simulink model "lab3_p6"  (R2020a)
settings: Solver=VariableStepAuto  StartTime=0.0  StopTime=stop_time  RelTol=1e-3
InitFcn:
  | % Read in the audio file
  | [input_wav_signal, Fs_in] = audioread('acoustic.wav');
  | % Fs_in = 11025, we need to convert this to Fs = 48k
  | 
  | % Convert the Sampling rate to 48 kHz
  | signal = resample(input_wav_signal, 48000, 11025);
  | Fs = 48000; % This is our desired sample rate that we converted to
  | Ts = 1/Fs; % The associated sample period
  | 
  | % Put signal inot a timeseries format
  | timevals = [0:length(signal)-1]*Ts;
  | input_signal = timeseries(signal,timevals);
  | 
  | % Set the simulation stop time
  | stop_time = length(signal)*Ts;
  | 
  | % Fixed-point precision we want the signal to be converted to
  | W_bits = 32;
  | F_bits = 28;
  | 
  | % Counter
  | max_counter_time = 5; % yime in seconds
  | max_reset_Nbits = ceil(log2(max_counter_time*Fs)); % size of counter
  | 
  | max_reset_time = 300; % time in milliseconds
  | max_reset_threshold = ceil(max_reset_time/1000 * Fs); % reset time in samples
  | 
  | % LED Persistence
  | LED_persistence_Nbits = 15;
  | LED_persistence_time = 100; %msec
  | LED_persistence = ceil(LED_persistence_time/1000 * Fs);
StopFcn:
  | y_out = output_signal.Data(:);
  | plot(y_out)
  | soundsc(y_out,Fs)
undefined symbols (not defined in the file): magnitude
libraries: hdlsllib x10, dspsrcs4 x2, simulink x1
settings Model: Creator=Owner  LastModifiedBy=Owner
settings DataIOCC: ReturnWorkspaceOutputs=off

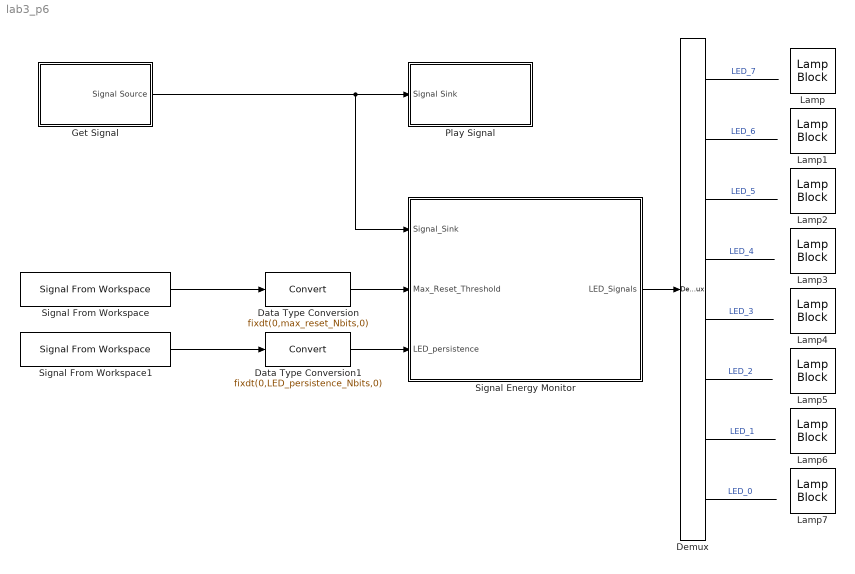
== system lab3_p6 ==
  Data Type Conversion : DataTypeConversion  OutDataTypeStr=fixdt(0,max_reset_Nbits,0)
  Data Type Conversion1 : DataTypeConversion  OutDataTypeStr=fixdt(0,LED_persistence_Nbits,0)
  Demux : Demux  Outputs=8
  Get Signal : Subsystem
  Lamp{,1..7} (8 alike) : LampBlock
  Play Signal : Subsystem
  Signal Energy Monitor : Subsystem
  Signal From Workspace : dspsrcs4/Signal From Workspace  X=max_reset_threshold  Ts=Ts  nsamps=1  OutputAfterFinalValue=Holding final value  ignoreOrWarnInputAndFrameLengths=off  OutputFrames=off
  Signal From Workspace1 : dspsrcs4/Signal From Workspace  X=LED_persistence  Ts=Ts  nsamps=1  OutputAfterFinalValue=Holding final value  ignoreOrWarnInputAndFrameLengths=off  OutputFrames=off
  wires:
  Get Signal/1(Signal Source) -> Signal Energy Monitor/1(Signal_Sink), Play Signal/1(Signal Sink)
  Signal Energy Monitor/1(LED_Signals) -> Demux/1
  Data Type Conversion/1 -> Signal Energy Monitor/2(Max_Reset_Threshold)
  Signal From Workspace/1 -> Data Type Conversion/1
  Demux/1 -> ?  "LED_7"
  Demux/2 -> ?  "LED_6"
  Demux/3 -> ?  "LED_5"
  Demux/4 -> ?  "LED_4"
  Demux/5 -> ?  "LED_3"
  Demux/6 -> ?  "LED_2"
  Demux/7 -> ?  "LED_1"
  Demux/8 -> ?  "LED_0"
  Signal From Workspace1/1 -> Data Type Conversion1/1
  Data Type Conversion1/1 -> Signal Energy Monitor/3(LED_persistence)

== system lab3_p6/Get Signal ==
  Data Type Conversion : DataTypeConversion  OutDataTypeStr=fixdt(1,W_bits,F_bits)
  From Workspace : FromWorkspace  VariableName=input_signal  SampleTime=Ts
  Signal Source : Outport
  wires:
  From Workspace/1 -> Data Type Conversion/1
  Data Type Conversion/1 -> Signal Source/1

== system lab3_p6/Play Signal ==
  Signal Sink : Inport
  Data Type Conversion1 : DataTypeConversion  OutDataTypeStr=double
  To Workspace : ToWorkspace  VariableName=output_signal  SaveFormat=Timeseries  SampleTime=-1
  wires:
  Data Type Conversion1/1 -> To Workspace/1
  Signal Sink/1 -> Data Type Conversion1/1

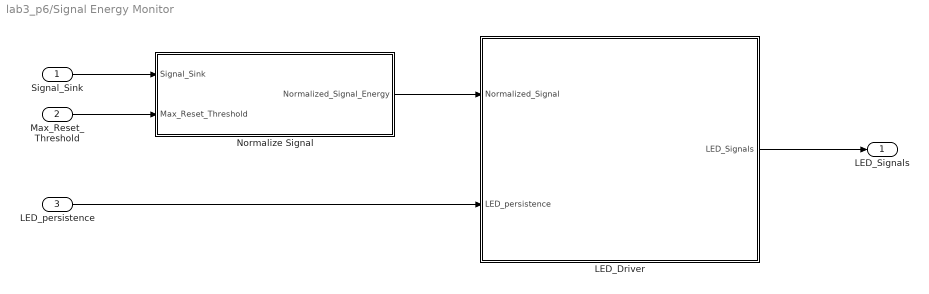
== system lab3_p6/Signal Energy Monitor ==
  Signal_Sink : Inport
  Max_Reset_Threshold : Inport  Port=2
  LED_persistence : Inport  Port=3
  LED_Driver : Subsystem
  Normalize Signal : Subsystem
  LED_Signals : Outport  VectorParamsAs1DForOutWhenUnconnected=off
  wires:
  Signal_Sink/1 -> Normalize Signal/1(Signal_Sink)
  Max_Reset_Threshold/1 -> Normalize Signal/2(Max_Reset_Threshold)
  Normalize Signal/1(Normalized_Signal_Energy) -> LED_Driver/1(Normalized_Signal)
  LED_Driver/1(LED_Signals) -> LED_Signals/1
  LED_persistence/1 -> LED_Driver/2(LED_persistence)

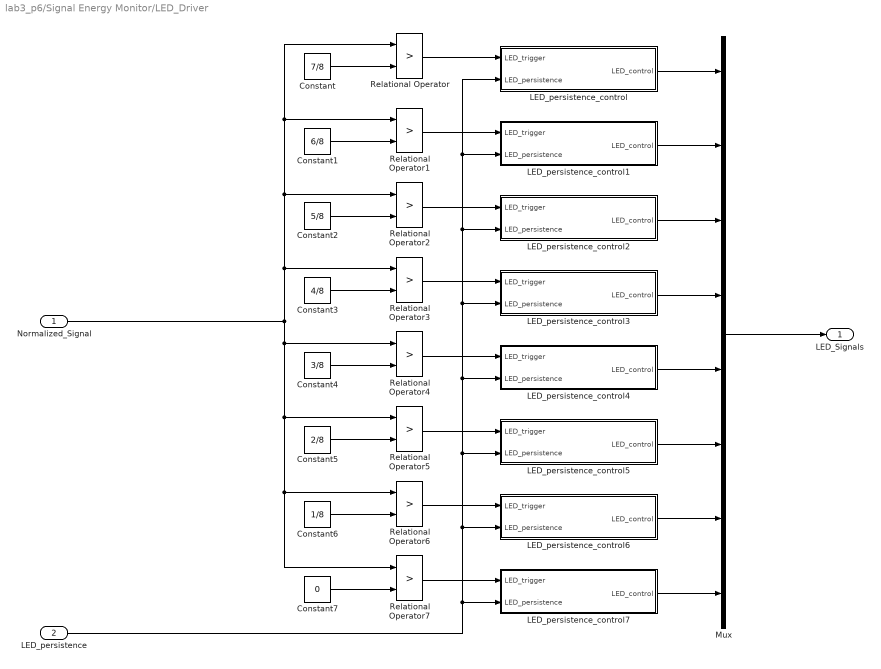
== system lab3_p6/Signal Energy Monitor/LED_Driver ==
  Normalized_Signal : Inport
  LED_persistence : Inport  Port=2
  Constant : Constant  Value=7/8  OutDataTypeStr=fixdt(1,W_bits,F_bits)  SampleTime=Ts
  Constant1 : Constant  Value=6/8  OutDataTypeStr=fixdt(1,W_bits,F_bits)  SampleTime=Ts
  Constant2 : Constant  Value=5/8  OutDataTypeStr=fixdt(1,W_bits,F_bits)  SampleTime=Ts
  Constant3 : Constant  Value=4/8  OutDataTypeStr=fixdt(1,W_bits,F_bits)  SampleTime=Ts
  Constant4 : Constant  Value=3/8  OutDataTypeStr=fixdt(1,W_bits,F_bits)  SampleTime=Ts
  Constant5 : Constant  Value=2/8  OutDataTypeStr=fixdt(1,W_bits,F_bits)  SampleTime=Ts
  Constant6 : Constant  Value=1/8  OutDataTypeStr=fixdt(1,W_bits,F_bits)  SampleTime=Ts
  Constant7 : Constant  Value=0  OutDataTypeStr=fixdt(1,W_bits,F_bits)  SampleTime=Ts
  LED_persistence_control : Subsystem
  LED_persistence_control1 : Subsystem
  LED_persistence_control2 : Subsystem
  LED_persistence_control3 : Subsystem
  LED_persistence_control4 : Subsystem
  LED_persistence_control5 : Subsystem
  LED_persistence_control6 : Subsystem
  LED_persistence_control7 : Subsystem
  Mux : Mux  Inputs=8
  Relational Operator{,1..7} (8 alike) : RelationalOperator  Operator=>  OutDataTypeStr=boolean  RndMeth=Nearest
  LED_Signals : Outport
  wires:
  Constant/1 -> Relational Operator/2
  Normalized_Signal/1 -> Relational Operator4/1, Relational Operator5/1, Relational Operator7/1, Relational Operator6/1, Relational Operator/1, Relational Operator1/1, Relational Operator2/1, Relational Operator3/1
  Constant1/1 -> Relational Operator1/2
  Constant2/1 -> Relational Operator2/2
  Constant3/1 -> Relational Operator3/2
  Constant4/1 -> Relational Operator4/2
  Constant5/1 -> Relational Operator5/2
  Constant6/1 -> Relational Operator6/2
  Constant7/1 -> Relational Operator7/2
  Mux/1 -> LED_Signals/1
  Relational Operator/1 -> LED_persistence_control/1(LED_trigger)
  LED_persistence_control/1(LED_control) -> Mux/1
  Relational Operator1/1 -> LED_persistence_control1/1(LED_trigger)
  Relational Operator2/1 -> LED_persistence_control2/1(LED_trigger)
  Relational Operator3/1 -> LED_persistence_control3/1(LED_trigger)
  Relational Operator4/1 -> LED_persistence_control4/1(LED_trigger)
  Relational Operator5/1 -> LED_persistence_control5/1(LED_trigger)
  LED_persistence/1 -> LED_persistence_control7/2(LED_persistence), LED_persistence_control6/2(LED_persistence), LED_persistence_control5/2(LED_persistence), LED_persistence_control4/2(LED_persistence), LED_persistence_control3/2(LED_persistence), LED_persistence_control2/2(LED_persistence), LED_persistence_control1/2(LED_persistence), LED_persistence_control/2(LED_persistence)
  Relational Operator6/1 -> LED_persistence_control6/1(LED_trigger)
  Relational Operator7/1 -> LED_persistence_control7/1(LED_trigger)
  LED_persistence_control7/1(LED_control) -> Mux/8
  LED_persistence_control6/1(LED_control) -> Mux/7
  LED_persistence_control5/1(LED_control) -> Mux/6
  LED_persistence_control4/1(LED_control) -> Mux/5
  LED_persistence_control3/1(LED_control) -> Mux/4
  LED_persistence_control2/1(LED_control) -> Mux/3
  LED_persistence_control1/1(LED_control) -> Mux/2

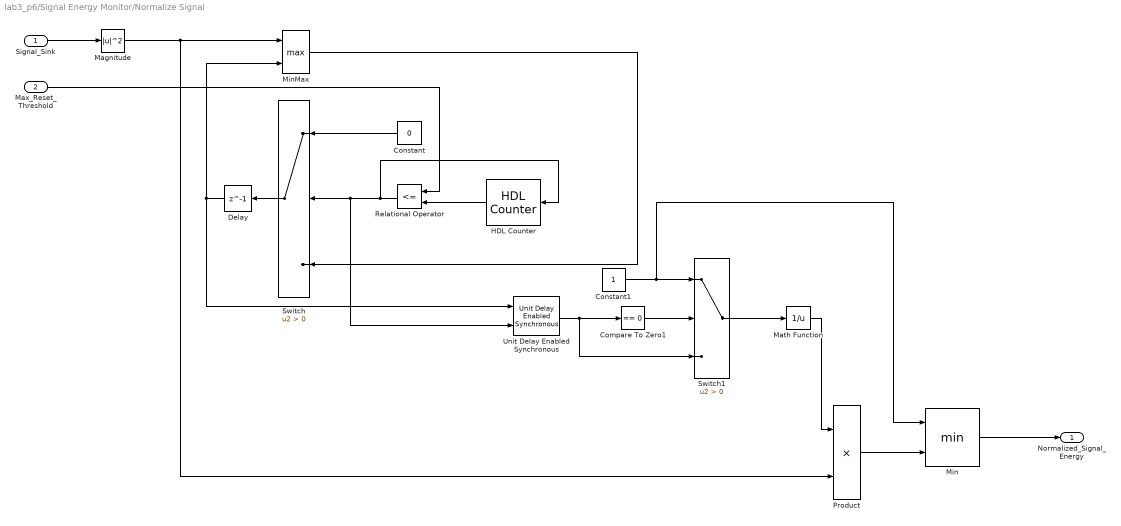
== system lab3_p6/Signal Energy Monitor/Normalize Signal ==
  Signal_Sink : Inport
  Max_Reset_Threshold : Inport  Port=2
  Compare To Zero1 : simulink/Logic and Bit Operations/Compare To Zero  relop===  OutDataTypeStr=boolean
  Constant : Constant  Value=0  OutDataTypeStr=fixdt(1,W_bits,F_bits)  SampleTime=Ts
  Constant1 : Constant  OutDataTypeStr=fixdt(1,W_bits,F_bits)  SampleTime=Ts
  Delay : Delay  DelayLength=1
  HDL Counter : hdlsllib/Sources/HDL Counter  CountType=Free running  CountInit=0  CountStep=1  CountMax=25  CountFromType=Initial value  CountFrom=0  CountResetPort=on  CountLoadPort=off  CountEnbPort=off  CountDirPort=off  CountDataType=Unsigned  CountWordLen=max_reset_Nbits  CountFracLen=0  CountSampTime=1
  Magnitude : Math  Operator=magnitude^2  SignedPower=on  RndMeth=Zero  SaturateOnIntegerOverflow=on
  Math Function : Math  Operator=reciprocal  OutDataTypeStr=fixdt(1,32,24)  SaturateOnIntegerOverflow=on
  Min : MinMax  Inputs=2  OutDataTypeStr=fixdt(1,W_bits,F_bits)
  MinMax : MinMax  Function=max  Inputs=2
  Product : Product  OutDataTypeStr=fixdt(1,W_bits,F_bits)
  Relational Operator : RelationalOperator  Operator=<=  OutDataTypeStr=boolean  RndMeth=Nearest
  Switch : Switch  Criteria=u2 > Threshold
  Switch1 : Switch  Criteria=u2 > Threshold
  Unit Delay Enabled Synchronous : hdlsllib/Discrete/Unit Delay Enabled Synchronous  InitialCondition=0.0  SampleTime=-1
      settings: SourceProductBaseCode=SL
  Normalized_Signal_Energy : Outport
  wires:
  Delay/1 -> MinMax/2, Unit Delay Enabled Synchronous/1
  Unit Delay Enabled Synchronous/1 -> Switch1/3, Compare To Zero1/1
  Min/1 -> Normalized_Signal_Energy/1
  Math Function/1 -> Product/1
  Relational Operator/1 -> HDL Counter/1, Unit Delay Enabled Synchronous/2, Switch/2
  Constant/1 -> Switch/1
  MinMax/1 -> Switch/3
  Constant1/1 -> Min/1, Switch1/1
  Compare To Zero1/1 -> Switch1/2
  Magnitude/1 -> Product/2, MinMax/1
  Switch/1 -> Delay/1
  Signal_Sink/1 -> Magnitude/1
  Switch1/1 -> Math Function/1
  Product/1 -> Min/2
  HDL Counter/1 -> Relational Operator/2
  Max_Reset_Threshold/1 -> Relational Operator/1

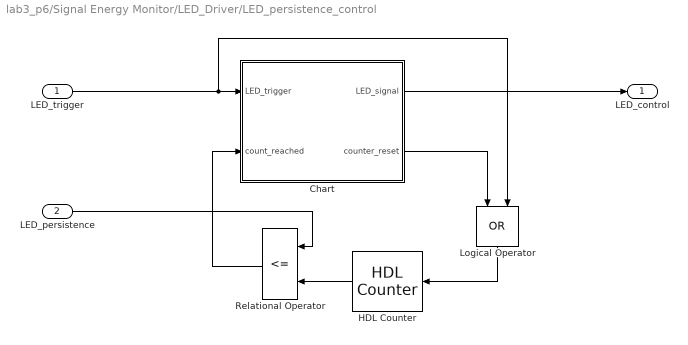
== system lab3_p6/Signal Energy Monitor/LED_Driver/LED_persistence_control ==
  LED_trigger : Inport
  LED_persistence : Inport  Port=2
  Chart : Stateflow chart  TreatAsAtomicUnit=on
  HDL Counter : hdlsllib/Sources/HDL Counter  CountType=Free running  CountInit=0  CountStep=1  CountMax=25  CountFromType=Initial value  CountFrom=0  CountResetPort=on  CountLoadPort=off  CountEnbPort=off  CountDirPort=off  CountDataType=Unsigned  CountWordLen=LED_persistence_Nbits  CountFracLen=0  CountSampTime=1
  Logical Operator : Logic  Operator=OR  AllPortsSameDT=off  OutDataTypeStr=boolean
  Relational Operator : RelationalOperator  Operator=<=  OutDataTypeStr=boolean  RndMeth=Nearest
  LED_control : Outport
  wires:
  LED_trigger/1 -> Logical Operator/2, Chart/1(LED_trigger)
  Logical Operator/1 -> HDL Counter/1
  Chart/2(counter_reset) -> Logical Operator/1
  LED_persistence/1 -> Relational Operator/1
  HDL Counter/1 -> Relational Operator/2
  Relational Operator/1 -> Chart/2(count_reached)
  Chart/1(LED_signal) -> LED_control/1

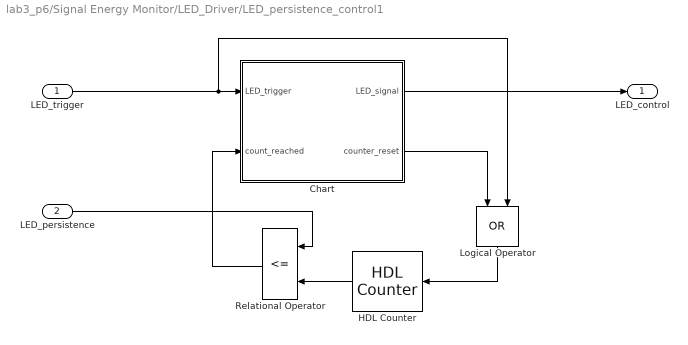
== system lab3_p6/Signal Energy Monitor/LED_Driver/LED_persistence_control1 ==
  LED_trigger : Inport
  LED_persistence : Inport  Port=2
  Chart : Stateflow chart  TreatAsAtomicUnit=on
  HDL Counter : hdlsllib/Sources/HDL Counter  CountType=Free running  CountInit=0  CountStep=1  CountMax=25  CountFromType=Initial value  CountFrom=0  CountResetPort=on  CountLoadPort=off  CountEnbPort=off  CountDirPort=off  CountDataType=Unsigned  CountWordLen=LED_persistence_Nbits  CountFracLen=0  CountSampTime=1
  Logical Operator : Logic  Operator=OR  AllPortsSameDT=off  OutDataTypeStr=boolean
  Relational Operator : RelationalOperator  Operator=<=  OutDataTypeStr=boolean  RndMeth=Nearest
  LED_control : Outport
  wires:
  LED_trigger/1 -> Logical Operator/2, Chart/1(LED_trigger)
  Logical Operator/1 -> HDL Counter/1
  Chart/2(counter_reset) -> Logical Operator/1
  LED_persistence/1 -> Relational Operator/1
  HDL Counter/1 -> Relational Operator/2
  Relational Operator/1 -> Chart/2(count_reached)
  Chart/1(LED_signal) -> LED_control/1

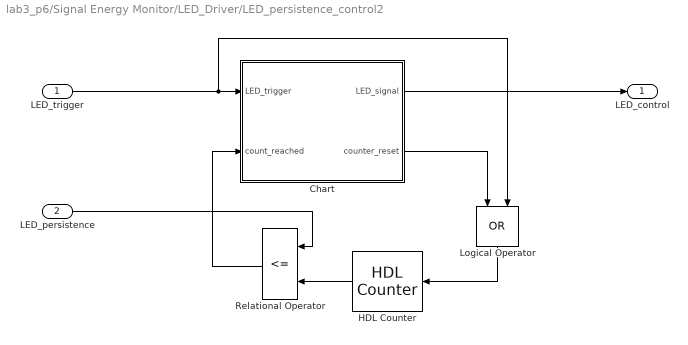
== system lab3_p6/Signal Energy Monitor/LED_Driver/LED_persistence_control2 ==
  LED_trigger : Inport
  LED_persistence : Inport  Port=2
  Chart : Stateflow chart  TreatAsAtomicUnit=on
  HDL Counter : hdlsllib/Sources/HDL Counter  CountType=Free running  CountInit=0  CountStep=1  CountMax=25  CountFromType=Initial value  CountFrom=0  CountResetPort=on  CountLoadPort=off  CountEnbPort=off  CountDirPort=off  CountDataType=Unsigned  CountWordLen=LED_persistence_Nbits  CountFracLen=0  CountSampTime=1
  Logical Operator : Logic  Operator=OR  AllPortsSameDT=off  OutDataTypeStr=boolean
  Relational Operator : RelationalOperator  Operator=<=  OutDataTypeStr=boolean  RndMeth=Nearest
  LED_control : Outport
  wires:
  LED_trigger/1 -> Logical Operator/2, Chart/1(LED_trigger)
  Logical Operator/1 -> HDL Counter/1
  Chart/2(counter_reset) -> Logical Operator/1
  LED_persistence/1 -> Relational Operator/1
  HDL Counter/1 -> Relational Operator/2
  Relational Operator/1 -> Chart/2(count_reached)
  Chart/1(LED_signal) -> LED_control/1

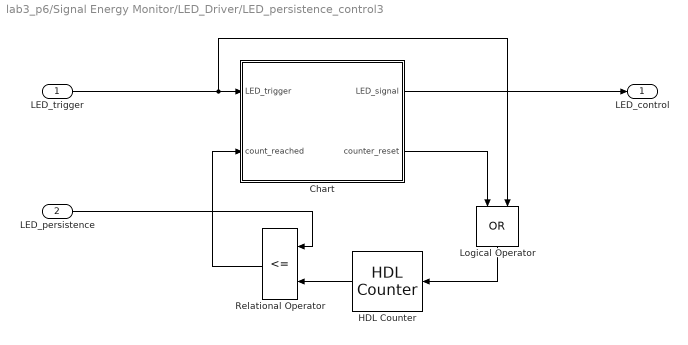
== system lab3_p6/Signal Energy Monitor/LED_Driver/LED_persistence_control3 ==
  LED_trigger : Inport
  LED_persistence : Inport  Port=2
  Chart : Stateflow chart  TreatAsAtomicUnit=on
  HDL Counter : hdlsllib/Sources/HDL Counter  CountType=Free running  CountInit=0  CountStep=1  CountMax=25  CountFromType=Initial value  CountFrom=0  CountResetPort=on  CountLoadPort=off  CountEnbPort=off  CountDirPort=off  CountDataType=Unsigned  CountWordLen=LED_persistence_Nbits  CountFracLen=0  CountSampTime=1
  Logical Operator : Logic  Operator=OR  AllPortsSameDT=off  OutDataTypeStr=boolean
  Relational Operator : RelationalOperator  Operator=<=  OutDataTypeStr=boolean  RndMeth=Nearest
  LED_control : Outport
  wires:
  LED_trigger/1 -> Logical Operator/2, Chart/1(LED_trigger)
  Logical Operator/1 -> HDL Counter/1
  Chart/2(counter_reset) -> Logical Operator/1
  LED_persistence/1 -> Relational Operator/1
  HDL Counter/1 -> Relational Operator/2
  Relational Operator/1 -> Chart/2(count_reached)
  Chart/1(LED_signal) -> LED_control/1

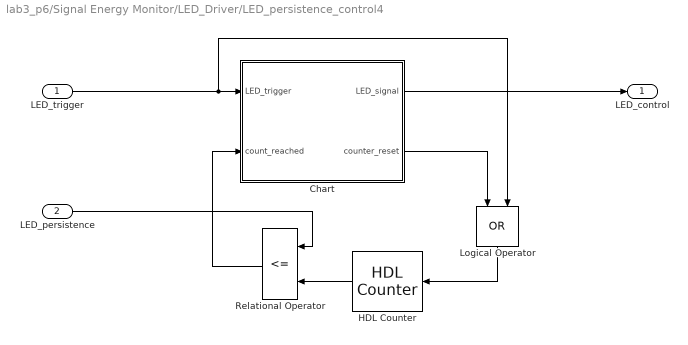
== system lab3_p6/Signal Energy Monitor/LED_Driver/LED_persistence_control4 ==
  LED_trigger : Inport
  LED_persistence : Inport  Port=2
  Chart : Stateflow chart  TreatAsAtomicUnit=on
  HDL Counter : hdlsllib/Sources/HDL Counter  CountType=Free running  CountInit=0  CountStep=1  CountMax=25  CountFromType=Initial value  CountFrom=0  CountResetPort=on  CountLoadPort=off  CountEnbPort=off  CountDirPort=off  CountDataType=Unsigned  CountWordLen=LED_persistence_Nbits  CountFracLen=0  CountSampTime=1
  Logical Operator : Logic  Operator=OR  AllPortsSameDT=off  OutDataTypeStr=boolean
  Relational Operator : RelationalOperator  Operator=<=  OutDataTypeStr=boolean  RndMeth=Nearest
  LED_control : Outport
  wires:
  LED_trigger/1 -> Logical Operator/2, Chart/1(LED_trigger)
  Logical Operator/1 -> HDL Counter/1
  Chart/2(counter_reset) -> Logical Operator/1
  LED_persistence/1 -> Relational Operator/1
  HDL Counter/1 -> Relational Operator/2
  Relational Operator/1 -> Chart/2(count_reached)
  Chart/1(LED_signal) -> LED_control/1

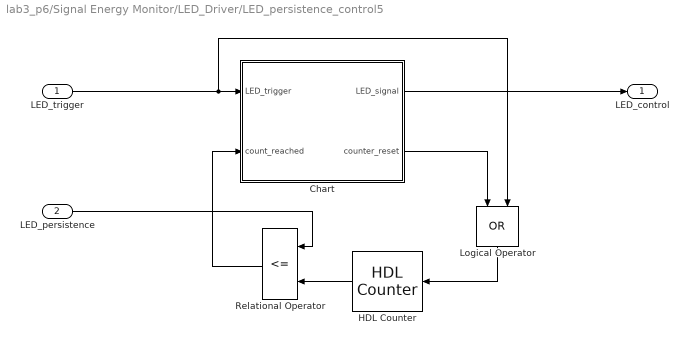
== system lab3_p6/Signal Energy Monitor/LED_Driver/LED_persistence_control5 ==
  LED_trigger : Inport
  LED_persistence : Inport  Port=2
  Chart : Stateflow chart  TreatAsAtomicUnit=on
  HDL Counter : hdlsllib/Sources/HDL Counter  CountType=Free running  CountInit=0  CountStep=1  CountMax=25  CountFromType=Initial value  CountFrom=0  CountResetPort=on  CountLoadPort=off  CountEnbPort=off  CountDirPort=off  CountDataType=Unsigned  CountWordLen=LED_persistence_Nbits  CountFracLen=0  CountSampTime=1
  Logical Operator : Logic  Operator=OR  AllPortsSameDT=off  OutDataTypeStr=boolean
  Relational Operator : RelationalOperator  Operator=<=  OutDataTypeStr=boolean  RndMeth=Nearest
  LED_control : Outport
  wires:
  LED_trigger/1 -> Logical Operator/2, Chart/1(LED_trigger)
  Logical Operator/1 -> HDL Counter/1
  Chart/2(counter_reset) -> Logical Operator/1
  LED_persistence/1 -> Relational Operator/1
  HDL Counter/1 -> Relational Operator/2
  Relational Operator/1 -> Chart/2(count_reached)
  Chart/1(LED_signal) -> LED_control/1

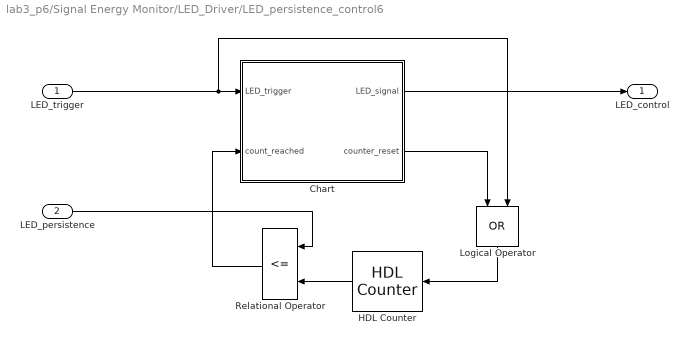
== system lab3_p6/Signal Energy Monitor/LED_Driver/LED_persistence_control6 ==
  LED_trigger : Inport
  LED_persistence : Inport  Port=2
  Chart : Stateflow chart  TreatAsAtomicUnit=on
  HDL Counter : hdlsllib/Sources/HDL Counter  CountType=Free running  CountInit=0  CountStep=1  CountMax=25  CountFromType=Initial value  CountFrom=0  CountResetPort=on  CountLoadPort=off  CountEnbPort=off  CountDirPort=off  CountDataType=Unsigned  CountWordLen=LED_persistence_Nbits  CountFracLen=0  CountSampTime=1
  Logical Operator : Logic  Operator=OR  AllPortsSameDT=off  OutDataTypeStr=boolean
  Relational Operator : RelationalOperator  Operator=<=  OutDataTypeStr=boolean  RndMeth=Nearest
  LED_control : Outport
  wires:
  LED_trigger/1 -> Logical Operator/2, Chart/1(LED_trigger)
  Logical Operator/1 -> HDL Counter/1
  Chart/2(counter_reset) -> Logical Operator/1
  LED_persistence/1 -> Relational Operator/1
  HDL Counter/1 -> Relational Operator/2
  Relational Operator/1 -> Chart/2(count_reached)
  Chart/1(LED_signal) -> LED_control/1

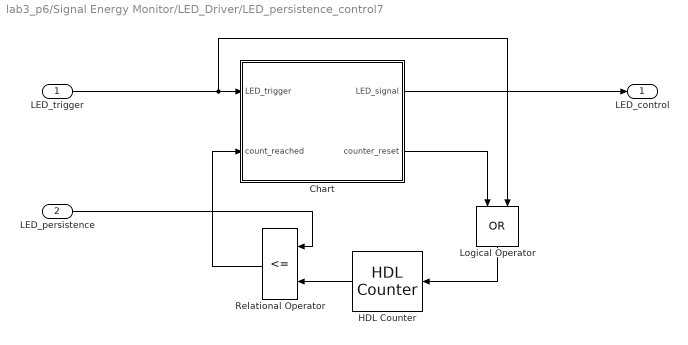
== system lab3_p6/Signal Energy Monitor/LED_Driver/LED_persistence_control7 ==
  LED_trigger : Inport
  LED_persistence : Inport  Port=2
  Chart : Stateflow chart  TreatAsAtomicUnit=on
  HDL Counter : hdlsllib/Sources/HDL Counter  CountType=Free running  CountInit=0  CountStep=1  CountMax=25  CountFromType=Initial value  CountFrom=0  CountResetPort=on  CountLoadPort=off  CountEnbPort=off  CountDirPort=off  CountDataType=Unsigned  CountWordLen=LED_persistence_Nbits  CountFracLen=0  CountSampTime=1
  Logical Operator : Logic  Operator=OR  AllPortsSameDT=off  OutDataTypeStr=boolean
  Relational Operator : RelationalOperator  Operator=<=  OutDataTypeStr=boolean  RndMeth=Nearest
  LED_control : Outport
  wires:
  LED_trigger/1 -> Logical Operator/2, Chart/1(LED_trigger)
  Logical Operator/1 -> HDL Counter/1
  Chart/2(counter_reset) -> Logical Operator/1
  LED_persistence/1 -> Relational Operator/1
  HDL Counter/1 -> Relational Operator/2
  Relational Operator/1 -> Chart/2(count_reached)
  Chart/1(LED_signal) -> LED_control/1

== stateflow chart lab3_p6/Signal Energy Monitor/LED_Driver/LED_persistence_control1/Chart ==
  state LED_off
    entry: LED_signal=false;
    entry: counter_reset=true;
  state LED_on
    entry: LED_signal=true;
    entry: counter_reset=false;
  (default) -> LED_off
  LED_off -> LED_on : [LED_trigger==1]
  LED_on -> LED_off : [count_reached==1]
  data: LED_trigger input; count_reached input; LED_signal output; counter_reset output

== stateflow chart lab3_p6/Signal Energy Monitor/LED_Driver/LED_persistence_control2/Chart ==
  state LED_off
    entry: LED_signal=false;
    entry: counter_reset=true;
  state LED_on
    entry: LED_signal=true;
    entry: counter_reset=false;
  (default) -> LED_off
  LED_off -> LED_on : [LED_trigger==1]
  LED_on -> LED_off : [count_reached==1]
  data: LED_trigger input; count_reached input; LED_signal output; counter_reset output

== stateflow chart lab3_p6/Signal Energy Monitor/LED_Driver/LED_persistence_control/Chart ==
  state LED_off
    entry: LED_signal=false;
    entry: counter_reset=true;
  state LED_on
    entry: LED_signal=true;
    entry: counter_reset=false;
  (default) -> LED_off
  LED_off -> LED_on : [LED_trigger==1]
  LED_on -> LED_off : [count_reached==1]
  data: LED_trigger input; count_reached input; LED_signal output; counter_reset output

== stateflow chart lab3_p6/Signal Energy Monitor/LED_Driver/LED_persistence_control3/Chart ==
  state LED_off
    entry: LED_signal=false;
    entry: counter_reset=true;
  state LED_on
    entry: LED_signal=true;
    entry: counter_reset=false;
  (default) -> LED_off
  LED_off -> LED_on : [LED_trigger==1]
  LED_on -> LED_off : [count_reached==1]
  data: LED_trigger input; count_reached input; LED_signal output; counter_reset output

== stateflow chart lab3_p6/Signal Energy Monitor/LED_Driver/LED_persistence_control4/Chart ==
  state LED_off
    entry: LED_signal=false;
    entry: counter_reset=true;
  state LED_on
    entry: LED_signal=true;
    entry: counter_reset=false;
  (default) -> LED_off
  LED_off -> LED_on : [LED_trigger==1]
  LED_on -> LED_off : [count_reached==1]
  data: LED_trigger input; count_reached input; LED_signal output; counter_reset output

== stateflow chart lab3_p6/Signal Energy Monitor/LED_Driver/LED_persistence_control5/Chart ==
  state LED_off
    entry: LED_signal=false;
    entry: counter_reset=true;
  state LED_on
    entry: LED_signal=true;
    entry: counter_reset=false;
  (default) -> LED_off
  LED_off -> LED_on : [LED_trigger==1]
  LED_on -> LED_off : [count_reached==1]
  data: LED_trigger input; count_reached input; LED_signal output; counter_reset output

== stateflow chart lab3_p6/Signal Energy Monitor/LED_Driver/LED_persistence_control6/Chart ==
  state LED_off
    entry: LED_signal=false;
    entry: counter_reset=true;
  state LED_on
    entry: LED_signal=true;
    entry: counter_reset=false;
  (default) -> LED_off
  LED_off -> LED_on : [LED_trigger==1]
  LED_on -> LED_off : [count_reached==1]
  data: LED_trigger input; count_reached input; LED_signal output; counter_reset output

== stateflow chart lab3_p6/Signal Energy Monitor/LED_Driver/LED_persistence_control7/Chart ==
  state LED_off
    entry: LED_signal=false;
    entry: counter_reset=true;
  state LED_on
    entry: LED_signal=true;
    entry: counter_reset=false;
  (default) -> LED_off
  LED_off -> LED_on : [LED_trigger==1]
  LED_on -> LED_off : [count_reached==1]
  data: LED_trigger input; count_reached input; LED_signal output; counter_reset output
